simulink model "fullcar"  (Simulink 9.1)
settings: Solver=ode45  StartTime=0.0  StopTime=100  RelTol=1e-3  EnableMultiTasking=on
undefined symbols (not defined in the file): a, b, c_1, c_2, c_3, c_4, c_p, c_t, F_1, F_2, F_3, F_4, I_x, I_y, k_1, k_2, k_3, k_4, k_p, k_t, M, m_1, m_2, m_3, m_4, m_p, sigbuilder_block, w, x_p, y_p
settings Model: Creator=Zhytenko_Olexandr  LastModifiedBy=Saurabh Suman
settings SolverCC: MaxConsecutiveZCs=auto
settings DataIOCC: SignalLoggingSaveFormat=ModelDataLogs
settings OptimizationCC: BlockReduction=off  OptimizeBlockIOStorage=off  BufferReuse=off  GlobalBufferReuse=off  ExpressionFolding=off  ExpressionDepthLimit=2147483647  LocalBlockOutputs=off  OptimizeDataStoreBuffers=off  BusAssignmentInplaceUpdate=off
settings DebuggingCC: FcnCallInpInsideContextMsg=warning  StateNameClashWarn=warning
settings GRTTargetCC: GeneratePreprocessorConditionals=Disable all

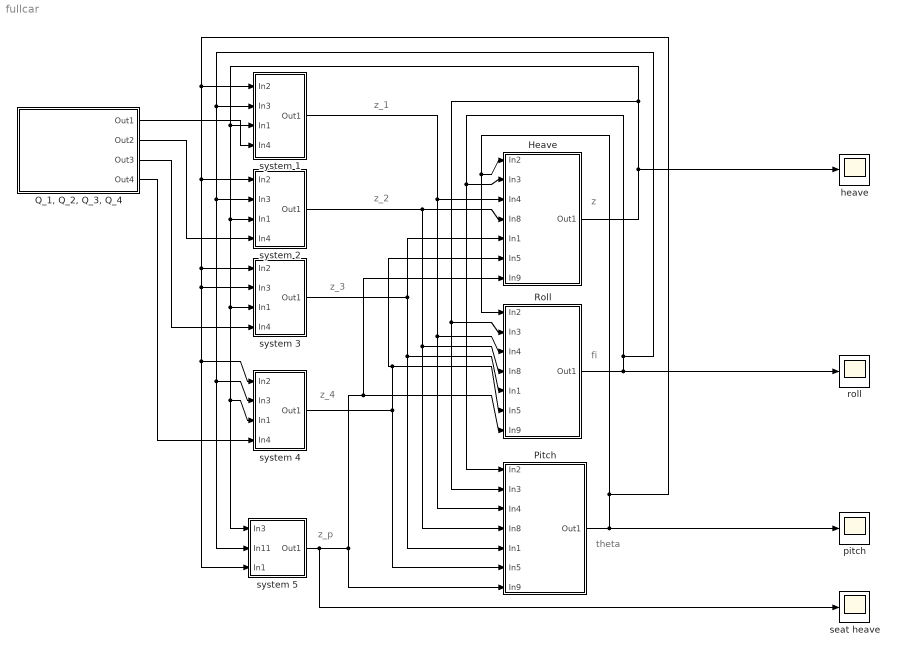
== system fullcar ==
  note: z
  note: fi
  note: theta
  note: z_p
  note: z_1
  note: z_2
  note: z_3
  note: z_4
  Heave : Subsystem
  Pitch : Subsystem
  "Q_1, Q_2, Q_3, Q_4" : Subsystem
  Roll : Subsystem
  heave : Scope
  pitch : Scope
  roll : Scope
  seat heave : Scope
  system 1 : Subsystem
  system 2 : Subsystem
  system 3 : Subsystem
  system 4 : Subsystem
  system 5 : Subsystem
  wires:
  Pitch/1(Out1) -> Heave/1(In2), Roll/1(In2), system 1/1(In2), system 2/1(In2), system 3/1(In2), system 3/2(In3), system 5/3(In1), system 4/1(In2), pitch/1
  Roll/1(Out1) -> Heave/2(In3), Pitch/1(In2), system 1/2(In3), system 2/2(In3), system 5/2(In11), system 4/2(In3), roll/1
  Heave/1(Out1) -> Roll/2(In3), Pitch/2(In3), system 1/3(In1), system 2/3(In1), system 3/3(In1), system 5/1(In3), system 4/3(In1), heave/1
  system 1/1(Out1) -> Heave/3(In4), Roll/3(In4), Pitch/3(In4)
  system 2/1(Out1) -> Heave/4(In8), Roll/4(In8), Pitch/4(In8)
  system 3/1(Out1) -> Heave/5(In1), Roll/5(In1), Pitch/5(In1)
  system 5/1(Out1) -> Heave/7(In9), Roll/7(In9), Pitch/7(In9), seat heave/1
  "Q_1, Q_2, Q_3, Q_4"/1(Out1) -> system 1/4(In4)
  "Q_1, Q_2, Q_3, Q_4"/2(Out2) -> system 2/4(In4)
  "Q_1, Q_2, Q_3, Q_4"/3(Out3) -> system 3/4(In4)
  "Q_1, Q_2, Q_3, Q_4"/4(Out4) -> system 4/4(In4)
  system 4/1(Out1) -> Heave/6(In5), Roll/6(In5), Pitch/6(In5)

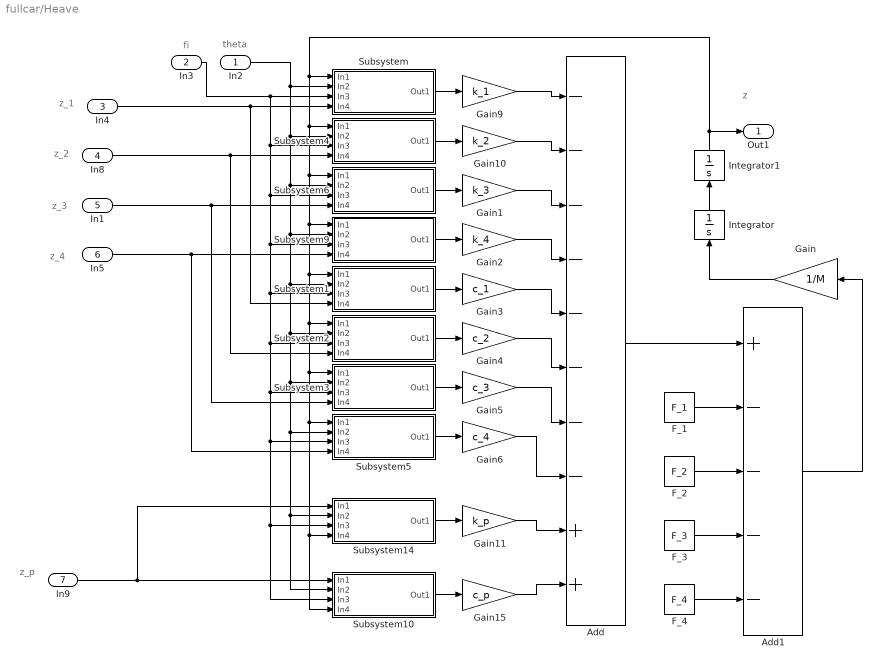
== system fullcar/Heave ==
  note: theta
  note: z
  note: fi
  note: z_1
  note: z_2
  note: z_3
  note: z_4
  note: z_p
  In2 : Inport
  In3 : Inport  Port=2
  In4 : Inport  Port=3
  In8 : Inport  Port=4
  In1 : Inport  Port=5
  In5 : Inport  Port=6
  In9 : Inport  Port=7
  Add : Sum  Inputs=--------++
  Add1 : Sum  Inputs=+----
  F_1 : Constant  Value=F_1
  F_2 : Constant  Value=F_2
  F_3 : Constant  Value=F_3
  F_4 : Constant  Value=F_4
  Gain : Gain  Gain=1/M
  Gain1 : Gain  Gain=k_3
  Gain10 : Gain  Gain=k_2
  Gain11 : Gain  Gain=k_p
  Gain15 : Gain  Gain=c_p
  Gain2 : Gain  Gain=k_4
  Gain3 : Gain  Gain=c_1
  Gain4 : Gain  Gain=c_2
  Gain5 : Gain  Gain=c_3
  Gain6 : Gain  Gain=c_4
  Gain9 : Gain  Gain=k_1
  Integrator : Integrator
  Integrator1 : Integrator
  Subsystem : Subsystem
  Subsystem1 : Subsystem
  Subsystem10 : Subsystem
  Subsystem14 : Subsystem
  Subsystem2 : Subsystem
  Subsystem3 : Subsystem
  Subsystem4 : Subsystem
  Subsystem5 : Subsystem
  Subsystem6 : Subsystem
  Subsystem9 : Subsystem
  Out1 : Outport
  wires:
  Gain10/1 -> Add/2
  Gain1/1 -> Add/3
  Gain2/1 -> Add/4
  Subsystem/1(Out1) -> Gain9/1
  Gain3/1 -> Add/5
  Gain4/1 -> Add/6
  Gain5/1 -> Add/7
  Subsystem1/1(Out1) -> Gain3/1
  Subsystem4/1(Out1) -> Gain10/1
  Subsystem2/1(Out1) -> Gain4/1
  Subsystem6/1(Out1) -> Gain1/1
  Subsystem3/1(Out1) -> Gain5/1
  Subsystem9/1(Out1) -> Gain2/1
  Subsystem5/1(Out1) -> Gain6/1
  Gain/1 -> Integrator/1
  Integrator/1 -> Integrator1/1
  Integrator1/1 -> Subsystem/1(In1), Subsystem4/1(In1), Subsystem6/1(In1), Subsystem9/1(In1), Subsystem1/1(In1), Subsystem2/1(In1), Subsystem3/1(In1), Subsystem5/1(In1), Subsystem10/4(In4), Subsystem14/4(In4), Out1/1
  Subsystem14/1(Out1) -> Gain11/1
  Subsystem10/1(Out1) -> Gain15/1
  In2/1 -> Subsystem/2(In2), Subsystem4/2(In2), Subsystem6/2(In2), Subsystem9/2(In2), Subsystem1/2(In2), Subsystem2/2(In2), Subsystem3/2(In2), Subsystem5/2(In2), Subsystem10/2(In2), Subsystem14/2(In2)
  In3/1 -> Subsystem/3(In3), Subsystem4/3(In3), Subsystem6/3(In3), Subsystem9/3(In3), Subsystem1/3(In3), Subsystem2/3(In3), Subsystem3/3(In3), Subsystem5/3(In3), Subsystem10/3(In3), Subsystem14/3(In3)
  In4/1 -> Subsystem/4(In4), Subsystem1/4(In4)
  In8/1 -> Subsystem4/4(In4), Subsystem2/4(In4)
  In1/1 -> Subsystem6/4(In4), Subsystem3/4(In4)
  In5/1 -> Subsystem9/4(In4), Subsystem5/4(In4)
  In9/1 -> Subsystem10/1(In1), Subsystem14/1(In1)
  Gain9/1 -> Add/1
  Gain15/1 -> Add/10
  Gain6/1 -> Add/8
  Gain11/1 -> Add/9
  Add/1 -> Add1/1
  F_1/1 -> Add1/2
  F_2/1 -> Add1/3
  F_3/1 -> Add1/4
  F_4/1 -> Add1/5
  Add1/1 -> Gain/1

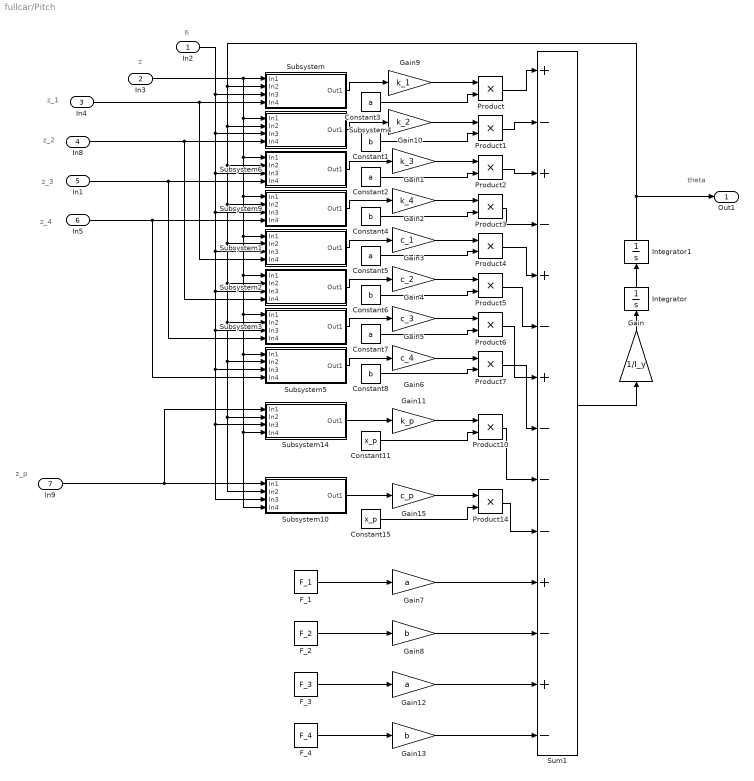
== system fullcar/Pitch ==
  note: fi
  note: theta
  note: z
  note: z_1
  note: z_2
  note: z_3
  note: z_4
  note: z_p
  In2 : Inport
  In3 : Inport  Port=2
  In4 : Inport  Port=3
  In8 : Inport  Port=4
  In1 : Inport  Port=5
  In5 : Inport  Port=6
  In9 : Inport  Port=7
  Constant{1,4,6,8} (4 alike) : Constant  Value=b
  Constant11 : Constant  Value=x_p
  Constant15 : Constant  Value=x_p
  Constant{2..3,5,7} (4 alike) : Constant  Value=a
  F_1 : Constant  Value=F_1
  F_2 : Constant  Value=F_2
  F_3 : Constant  Value=F_3
  F_4 : Constant  Value=F_4
  Gain : Gain  Gain=1/I_y
  Gain1 : Gain  Gain=k_3
  Gain10 : Gain  Gain=k_2
  Gain11 : Gain  Gain=k_p
  Gain12 : Gain  Gain=a
  Gain13 : Gain  Gain=b
  Gain15 : Gain  Gain=c_p
  Gain2 : Gain  Gain=k_4
  Gain3 : Gain  Gain=c_1
  Gain4 : Gain  Gain=c_2
  Gain5 : Gain  Gain=c_3
  Gain6 : Gain  Gain=c_4
  Gain7 : Gain  Gain=a
  Gain8 : Gain  Gain=b
  Gain9 : Gain  Gain=k_1
  Integrator : Integrator
  Integrator1 : Integrator
  Product{,1..7,10,14} (10 alike) : Product  RndMeth=Zero
  Subsystem : Subsystem
  Subsystem1 : Subsystem
  Subsystem10 : Subsystem
  Subsystem14 : Subsystem
  Subsystem2 : Subsystem
  Subsystem3 : Subsystem
  Subsystem4 : Subsystem
  Subsystem5 : Subsystem
  Subsystem6 : Subsystem
  Subsystem9 : Subsystem
  Sum1 : Sum  Inputs=+-+-+-+---+-+-
  Out1 : Outport
  wires:
  In3/1 -> Subsystem5/1(In1), Subsystem10/4(In4), Subsystem14/4(In4), Subsystem3/1(In1), Subsystem2/1(In1), Subsystem1/1(In1), Subsystem9/1(In1), Subsystem6/1(In1), Subsystem4/1(In1), Subsystem/1(In1)
  Constant15/1 -> Product14/2
  Gain15/1 -> Product14/1
  Constant11/1 -> Product10/2
  Gain11/1 -> Product10/1
  Constant8/1 -> Product7/2
  Subsystem5/1(Out1) -> Gain6/1
  Gain6/1 -> Product7/1
  Constant7/1 -> Product6/2
  Subsystem3/1(Out1) -> Gain5/1
  Gain5/1 -> Product6/1
  Constant6/1 -> Product5/2
  Subsystem2/1(Out1) -> Gain4/1
  Gain4/1 -> Product5/1
  Constant5/1 -> Product4/2
  Subsystem1/1(Out1) -> Gain3/1
  Gain3/1 -> Product4/1
  Constant4/1 -> Product3/2
  Subsystem9/1(Out1) -> Gain2/1
  Gain2/1 -> Product3/1
  Constant2/1 -> Product2/2
  Gain1/1 -> Product2/1
  Constant1/1 -> Product1/2
  Gain10/1 -> Product1/1
  Constant3/1 -> Product/2
  Gain9/1 -> Product/1
  Subsystem/1(Out1) -> Gain9/1
  Subsystem4/1(Out1) -> Gain10/1
  Subsystem6/1(Out1) -> Gain1/1
  Gain/1 -> Integrator/1
  Integrator/1 -> Integrator1/1
  Integrator1/1 -> Out1/1, Subsystem/2(In2), Subsystem4/2(In2), Subsystem6/2(In2), Subsystem9/2(In2), Subsystem1/2(In2), Subsystem2/2(In2), Subsystem3/2(In2), Subsystem5/2(In2), Subsystem10/2(In2), Subsystem14/2(In2)
  Subsystem14/1(Out1) -> Gain11/1
  Subsystem10/1(Out1) -> Gain15/1
  In4/1 -> Subsystem/4(In4), Subsystem1/4(In4)
  In8/1 -> Subsystem4/4(In4), Subsystem2/4(In4)
  In1/1 -> Subsystem6/4(In4), Subsystem3/4(In4)
  In5/1 -> Subsystem9/4(In4), Subsystem5/4(In4)
  In9/1 -> Subsystem10/1(In1), Subsystem14/1(In1)
  In2/1 -> Subsystem/3(In3), Subsystem4/3(In3), Subsystem6/3(In3), Subsystem9/3(In3), Subsystem1/3(In3), Subsystem2/3(In3), Subsystem3/3(In3), Subsystem5/3(In3), Subsystem10/3(In3), Subsystem14/3(In3)
  Product/1 -> Sum1/1
  Product1/1 -> Sum1/2
  Product2/1 -> Sum1/3
  Product3/1 -> Sum1/4
  Product4/1 -> Sum1/5
  Product5/1 -> Sum1/6
  Product6/1 -> Sum1/7
  Product7/1 -> Sum1/8
  Product10/1 -> Sum1/9
  Product14/1 -> Sum1/10
  F_1/1 -> Gain7/1
  F_2/1 -> Gain8/1
  F_3/1 -> Gain12/1
  F_4/1 -> Gain13/1
  Gain7/1 -> Sum1/11
  Gain8/1 -> Sum1/12
  Gain12/1 -> Sum1/13
  Gain13/1 -> Sum1/14
  Sum1/1 -> Gain/1

== system fullcar/Q_1, Q_2, Q_3, Q_4 ==
  note: Q_1
  note: Q_2
  note: Q_3
  note: Q_4
  Signal Builder : Subsystem  Tag=STV Subsys  LoadFcn=sigbuilder_block('load');  StartFcn=sigbuilder_block('start');  StopFcn=sigbuilder_block('stop');  ClipboardFcn=sigbuilder_block('clipboard');  mask(Sigbuilder block){tuvar=[0:10]}
      mask help: Create and generate interchangeable groups of signals whose waveforms are piecewise linear.
      mask init:
      | if ~strcmp(get_param(bdroot(gcbh),'SimulationStatus'),'stopped') tuvar = sigbuilder_block('maskInit'); end
      settings: CopyFcn=sigbuilder_block('copy');  DeleteFcn=sigbuilder_block('delete');  ModelCloseFcn=sigbuilder_block('modelClose');  PreSaveFcn=sigbuilder_block('preSave');  PauseFcn=sigbuilder_block('pause')  ContinueFcn=sigbuilder_block('continue')  NameChangeFcn=sigbuilder_block('namechange');  OpenFcn=sigbuilder_block('open',[437.25 118.5 550.5 394.5 ]);  CloseFcn=sigbuilder_block('close');
      mask Display: plot(0, 0, 100, 100,[2, 2, 32, 32, 2], [68, 8, 8, 68, 68],[32, 2], [38, 38], [32, 19, 2],[53, 60, 44], [32, 17, 17, 2],[16, 16, 31, 31]);txt = getActiveGroup(gcbh);text(2, 100, txt,'verticalAlignment', 'top');
  Transport Delay1 : TransportDelay  DelayTime=0.27
  Transport Delay2 : TransportDelay  DelayTime=0.27
  Out1 : Outport
  Out2 : Outport  Port=2
  Out3 : Outport  Port=3
  Out4 : Outport  Port=4
  wires:
  Signal Builder/1(Signal 1) -> Out1/1, Transport Delay1/1, Out3/1, Transport Delay2/1
  Transport Delay1/1 -> Out2/1
  Transport Delay2/1 -> Out4/1

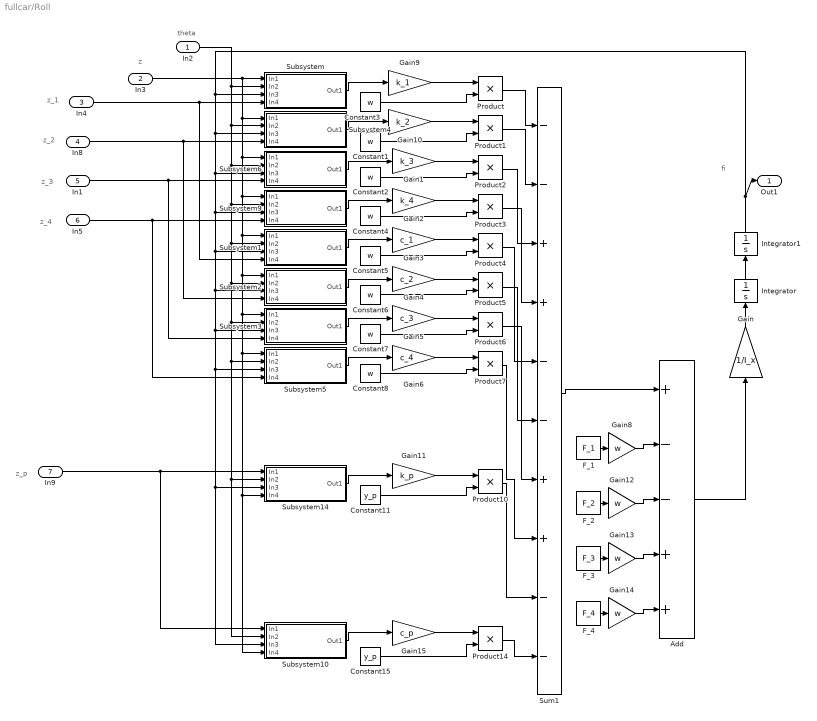
== system fullcar/Roll ==
  note: z_p
  note: z_4
  note: z_3
  note: z_2
  note: z_1
  note: z
  note: fi
  note: theta
  In2 : Inport
  In3 : Inport  Port=2
  In4 : Inport  Port=3
  In8 : Inport  Port=4
  In1 : Inport  Port=5
  In5 : Inport  Port=6
  In9 : Inport  Port=7
  Add : Sum  Inputs=+--++
  Constant{1..8} (8 alike) : Constant  Value=w
  Constant11 : Constant  Value=y_p
  Constant15 : Constant  Value=y_p
  F_1 : Constant  Value=F_1
  F_2 : Constant  Value=F_2
  F_3 : Constant  Value=F_3
  F_4 : Constant  Value=F_4
  Gain : Gain  Gain=1/I_x
  Gain1 : Gain  Gain=k_3
  Gain10 : Gain  Gain=k_2
  Gain11 : Gain  Gain=k_p
  Gain{8,12..14} (4 alike) : Gain  Gain=w
  Gain15 : Gain  Gain=c_p
  Gain2 : Gain  Gain=k_4
  Gain3 : Gain  Gain=c_1
  Gain4 : Gain  Gain=c_2
  Gain5 : Gain  Gain=c_3
  Gain6 : Gain  Gain=c_4
  Gain9 : Gain  Gain=k_1
  Integrator : Integrator  IgnoreLimit=on
  Integrator1 : Integrator
  Product{,1..7,10,14} (10 alike) : Product  RndMeth=Zero
  Subsystem : Subsystem
  Subsystem1 : Subsystem
  Subsystem10 : Subsystem
  Subsystem14 : Subsystem
  Subsystem2 : Subsystem
  Subsystem3 : Subsystem
  Subsystem4 : Subsystem
  Subsystem5 : Subsystem
  Subsystem6 : Subsystem
  Subsystem9 : Subsystem
  Sum1 : Sum  Inputs=--++--++--
  Out1 : Outport
  wires:
  In9/1 -> Subsystem10/1(In1), Subsystem14/1(In1)
  In5/1 -> Subsystem5/4(In4), Subsystem9/4(In4)
  In1/1 -> Subsystem3/4(In4), Subsystem6/4(In4)
  In8/1 -> Subsystem2/4(In4), Subsystem4/4(In4)
  In4/1 -> Subsystem1/4(In4), Subsystem/4(In4)
  In2/1 -> Subsystem5/2(In2), Subsystem14/2(In2), Subsystem10/2(In2), Subsystem3/2(In2), Subsystem2/2(In2), Subsystem1/2(In2), Subsystem9/2(In2), Subsystem6/2(In2), Subsystem4/2(In2), Subsystem/2(In2)
  Subsystem10/1(Out1) -> Gain15/1
  Subsystem14/1(Out1) -> Gain11/1
  Integrator1/1 -> Out1/1, Subsystem/3(In3), Subsystem4/3(In3), Subsystem6/3(In3), Subsystem9/3(In3), Subsystem1/3(In3), Subsystem2/3(In3), Subsystem3/3(In3), Subsystem5/3(In3), Subsystem14/3(In3), Subsystem10/3(In3)
  Integrator/1 -> Integrator1/1
  Gain/1 -> Integrator/1
  Subsystem6/1(Out1) -> Gain1/1
  Subsystem4/1(Out1) -> Gain10/1
  Subsystem/1(Out1) -> Gain9/1
  Product/1 -> Sum1/1
  Product1/1 -> Sum1/2
  Product2/1 -> Sum1/3
  Product3/1 -> Sum1/4
  Product4/1 -> Sum1/5
  Product5/1 -> Sum1/6
  Gain9/1 -> Product/1
  Constant3/1 -> Product/2
  Gain10/1 -> Product1/1
  Constant1/1 -> Product1/2
  Gain1/1 -> Product2/1
  Constant2/1 -> Product2/2
  Gain2/1 -> Product3/1
  Subsystem9/1(Out1) -> Gain2/1
  Constant4/1 -> Product3/2
  Gain3/1 -> Product4/1
  Subsystem1/1(Out1) -> Gain3/1
  Constant5/1 -> Product4/2
  Gain4/1 -> Product5/1
  Subsystem2/1(Out1) -> Gain4/1
  Constant6/1 -> Product5/2
  Gain5/1 -> Product6/1
  Subsystem3/1(Out1) -> Gain5/1
  Constant7/1 -> Product6/2
  Gain6/1 -> Product7/1
  Subsystem5/1(Out1) -> Gain6/1
  Constant8/1 -> Product7/2
  Gain11/1 -> Product10/1
  Constant11/1 -> Product10/2
  Gain15/1 -> Product14/1
  Constant15/1 -> Product14/2
  In3/1 -> Subsystem/1(In1), Subsystem4/1(In1), Subsystem6/1(In1), Subsystem9/1(In1), Subsystem1/1(In1), Subsystem2/1(In1), Subsystem3/1(In1), Subsystem5/1(In1), Subsystem14/4(In4), Subsystem10/4(In4)
  Sum1/1 -> Add/1
  Add/1 -> Gain/1
  F_1/1 -> Gain8/1
  Gain8/1 -> Add/2
  F_2/1 -> Gain12/1
  Gain12/1 -> Add/3
  F_3/1 -> Gain13/1
  Gain13/1 -> Add/4
  F_4/1 -> Gain14/1
  Gain14/1 -> Add/5
  Product6/1 -> Sum1/7
  Product7/1 -> Sum1/8
  Product10/1 -> Sum1/9
  Product14/1 -> Sum1/10

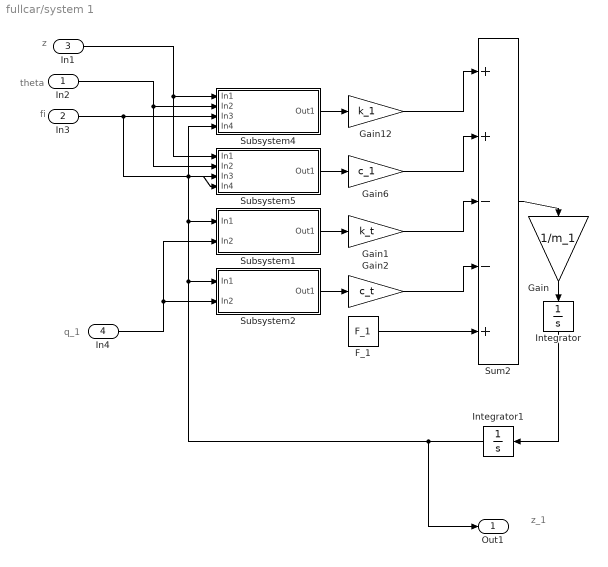
== system fullcar/system 1 ==
  note: fi
  note: z_1
  note: theta
  note: z
  note: q_1
  In2 : Inport
  In3 : Inport  Port=2
  In1 : Inport  Port=3
  In4 : Inport  Port=4
  F_1 : Constant  Value=F_1
  Gain : Gain  Gain=1/m_1
  Gain1 : Gain  Gain=k_t
  Gain12 : Gain  Gain=k_1
  Gain2 : Gain  Gain=c_t
  Gain6 : Gain  Gain=c_1
  Integrator : Integrator
  Integrator1 : Integrator
  Subsystem1 : Subsystem
  Subsystem2 : Subsystem
  Subsystem4 : Subsystem
  Subsystem5 : Subsystem
  Sum2 : Sum  Inputs=++--+
  Out1 : Outport
  wires:
  In3/1 -> Subsystem4/3(In3), Subsystem5/3(In3)
  In2/1 -> Subsystem4/2(In2), Subsystem5/2(In2)
  Integrator/1 -> Integrator1/1
  Gain/1 -> Integrator/1
  Gain6/1 -> Sum2/2
  Gain12/1 -> Sum2/1
  In1/1 -> Subsystem4/1(In1), Subsystem5/1(In1)
  Gain1/1 -> Sum2/3
  Gain2/1 -> Sum2/4
  Subsystem1/1(Out1) -> Gain1/1
  Subsystem2/1(Out1) -> Gain2/1
  Sum2/1 -> Gain/1
  Integrator1/1 -> Subsystem4/4(In4), Subsystem5/4(In4), Subsystem1/1(In1), Subsystem2/1(In1), Out1/1
  In4/1 -> Subsystem2/2(In2), Subsystem1/2(In2)
  Subsystem4/1(Out1) -> Gain12/1
  Subsystem5/1(Out1) -> Gain6/1
  F_1/1 -> Sum2/5

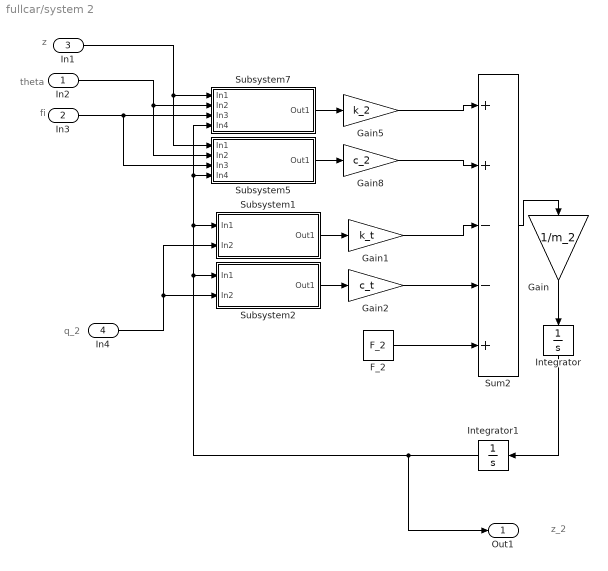
== system fullcar/system 2 ==
  note: q_2
  note: z
  note: theta
  note: z_2
  note: fi
  In2 : Inport
  In3 : Inport  Port=2
  In1 : Inport  Port=3
  In4 : Inport  Port=4
  F_2 : Constant  Value=F_2
  Gain : Gain  Gain=1/m_2
  Gain1 : Gain  Gain=k_t
  Gain2 : Gain  Gain=c_t
  Gain5 : Gain  Gain=k_2
  Gain8 : Gain  Gain=c_2
  Integrator : Integrator
  Integrator1 : Integrator
  Subsystem1 : Subsystem
  Subsystem2 : Subsystem
  Subsystem5 : Subsystem
  Subsystem7 : Subsystem
  Sum2 : Sum  Inputs=++--+
  Out1 : Outport
  wires:
  In4/1 -> Subsystem2/2(In2), Subsystem1/2(In2)
  Integrator1/1 -> Subsystem7/4(In4), Subsystem5/4(In4), Subsystem1/1(In1), Subsystem2/1(In1), Out1/1
  Subsystem2/1(Out1) -> Gain2/1
  Subsystem1/1(Out1) -> Gain1/1
  Gain2/1 -> Sum2/4
  Gain1/1 -> Sum2/3
  In1/1 -> Subsystem7/1(In1), Subsystem5/1(In1)
  Gain5/1 -> Sum2/1
  Gain8/1 -> Sum2/2
  In2/1 -> Subsystem7/2(In2), Subsystem5/2(In2)
  In3/1 -> Subsystem7/3(In3), Subsystem5/3(In3)
  Subsystem7/1(Out1) -> Gain5/1
  Subsystem5/1(Out1) -> Gain8/1
  F_2/1 -> Sum2/5
  Integrator/1 -> Integrator1/1
  Gain/1 -> Integrator/1
  Sum2/1 -> Gain/1

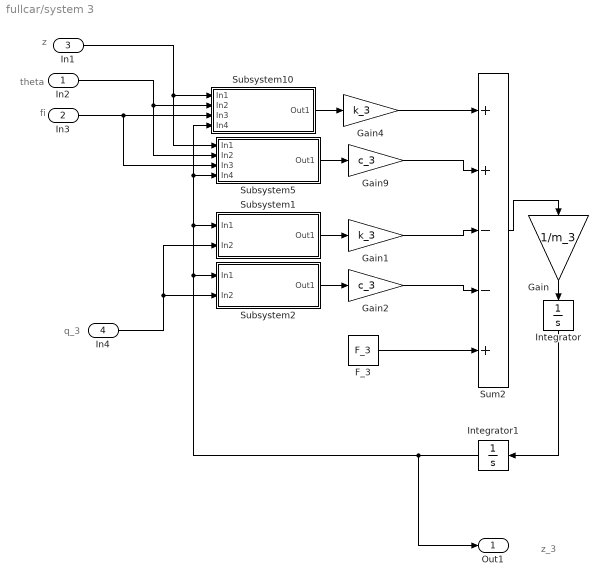
== system fullcar/system 3 ==
  note: fi
  note: z_3
  note: theta
  note: z
  note: q_3
  In2 : Inport
  In3 : Inport  Port=2
  In1 : Inport  Port=3
  In4 : Inport  Port=4
  F_3 : Constant  Value=F_3
  Gain : Gain  Gain=1/m_3
  Gain1 : Gain  Gain=k_3
  Gain2 : Gain  Gain=c_3
  Gain4 : Gain  Gain=k_3
  Gain9 : Gain  Gain=c_3
  Integrator : Integrator
  Integrator1 : Integrator
  Subsystem1 : Subsystem
  Subsystem10 : Subsystem
  Subsystem2 : Subsystem
  Subsystem5 : Subsystem
  Sum2 : Sum  Inputs=++--+
  Out1 : Outport
  wires:
  In3/1 -> Subsystem10/3(In3), Subsystem5/3(In3)
  In2/1 -> Subsystem10/2(In2), Subsystem5/2(In2)
  Integrator/1 -> Integrator1/1
  Gain/1 -> Integrator/1
  Gain9/1 -> Sum2/2
  Gain4/1 -> Sum2/1
  In1/1 -> Subsystem10/1(In1), Subsystem5/1(In1)
  Gain1/1 -> Sum2/3
  Gain2/1 -> Sum2/4
  Subsystem1/1(Out1) -> Gain1/1
  Subsystem2/1(Out1) -> Gain2/1
  Sum2/1 -> Gain/1
  Integrator1/1 -> Subsystem2/1(In1), Subsystem1/1(In1), Subsystem10/4(In4), Subsystem5/4(In4), Out1/1
  In4/1 -> Subsystem1/2(In2), Subsystem2/2(In2)
  Subsystem10/1(Out1) -> Gain4/1
  Subsystem5/1(Out1) -> Gain9/1
  F_3/1 -> Sum2/5

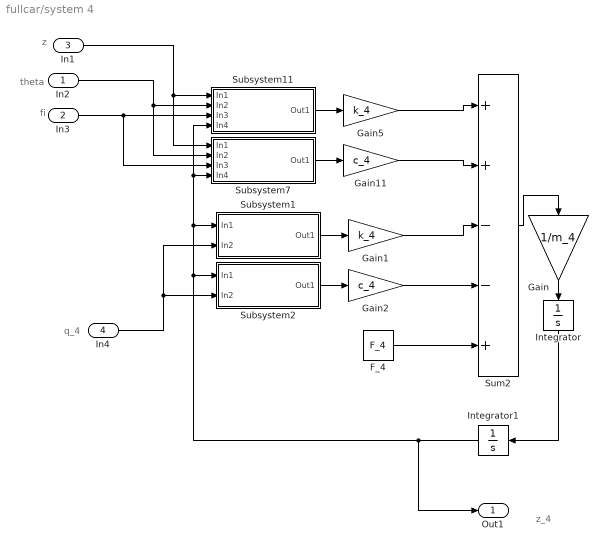
== system fullcar/system 4 ==
  note: q_4
  note: z
  note: theta
  note: z_4
  note: fi
  In2 : Inport
  In3 : Inport  Port=2
  In1 : Inport  Port=3
  In4 : Inport  Port=4
  F_4 : Constant  Value=F_4
  Gain : Gain  Gain=1/m_4
  Gain1 : Gain  Gain=k_4
  Gain11 : Gain  Gain=c_4
  Gain2 : Gain  Gain=c_4
  Gain5 : Gain  Gain=k_4
  Integrator : Integrator
  Integrator1 : Integrator
  Subsystem1 : Subsystem
  Subsystem11 : Subsystem
  Subsystem2 : Subsystem
  Subsystem7 : Subsystem
  Sum2 : Sum  Inputs=++--+
  Out1 : Outport
  wires:
  In4/1 -> Subsystem2/2(In2), Subsystem1/2(In2)
  Integrator1/1 -> Subsystem11/4(In4), Subsystem7/4(In4), Subsystem1/1(In1), Subsystem2/1(In1), Out1/1
  Sum2/1 -> Gain/1
  Subsystem2/1(Out1) -> Gain2/1
  Subsystem1/1(Out1) -> Gain1/1
  Gain2/1 -> Sum2/4
  Gain1/1 -> Sum2/3
  In1/1 -> Subsystem11/1(In1), Subsystem7/1(In1)
  Gain5/1 -> Sum2/1
  Gain11/1 -> Sum2/2
  Gain/1 -> Integrator/1
  Integrator/1 -> Integrator1/1
  In2/1 -> Subsystem11/2(In2), Subsystem7/2(In2)
  In3/1 -> Subsystem11/3(In3), Subsystem7/3(In3)
  Subsystem11/1(Out1) -> Gain5/1
  Subsystem7/1(Out1) -> Gain11/1
  F_4/1 -> Sum2/5

== system fullcar/system 5 ==
  note: fi
  note: z_3
  note: z
  note: theta
  In3 : Inport
  In11 : Inport  Port=2
  In1 : Inport  Port=3
  Gain : Gain  Gain=1/m_p
  Gain3 : Gain  Gain=k_p
  Gain4 : Gain  Gain=c_p
  Integrator : Integrator
  Integrator1 : Integrator
  Subsystem2 : Subsystem
  Subsystem3 : Subsystem
  Sum : Sum  Inputs=--
  Out1 : Outport
  wires:
  Integrator/1 -> Integrator1/1
  Gain/1 -> Integrator/1
  Sum/1 -> Gain/1
  Gain4/1 -> Sum/2
  Gain3/1 -> Sum/1
  In1/1 -> Subsystem2/2(In2), Subsystem3/2(In2)
  Integrator1/1 -> Out1/1, Subsystem2/1(In1), Subsystem3/1(In1)
  Subsystem2/1(Out1) -> Gain3/1
  Subsystem3/1(Out1) -> Gain4/1
  In11/1 -> Subsystem2/3(In3), Subsystem3/3(In3)
  In3/1 -> Subsystem2/4(In4), Subsystem3/4(In4)

== system fullcar/Heave/Subsystem ==
  note: z
  note: theta
  note: fi
  note: z_1
  In1 : Inport
  In2 : Inport  Port=2
  In3 : Inport  Port=3
  In4 : Inport  Port=4
  Constant : Constant  Value=a
  Constant1 : Constant  Value=w
  Product : Product  RndMeth=Zero
  Product1 : Product  RndMeth=Zero
  Sum : Sum  Inputs=+-+
  Sum1 : Sum  Inputs=+-
  Out1 : Outport
  wires:
  Sum1/1 -> Out1/1
  Sum/1 -> Sum1/1
  In4/1 -> Sum1/2
  In1/1 -> Sum/1
  In2/1 -> Product/1
  Constant/1 -> Product/2
  Product/1 -> Sum/2
  In3/1 -> Product1/1
  Constant1/1 -> Product1/2
  Product1/1 -> Sum/3

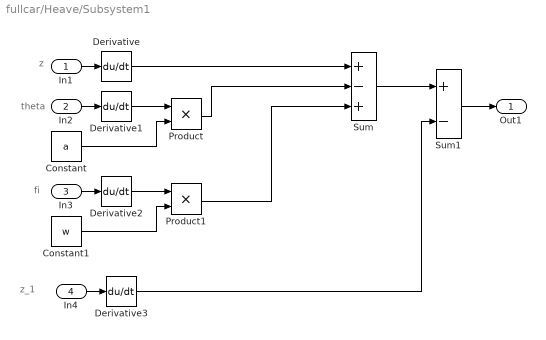
== system fullcar/Heave/Subsystem1 ==
  note: z_1
  note: fi
  note: theta
  note: z
  In1 : Inport
  In2 : Inport  Port=2
  In3 : Inport  Port=3
  In4 : Inport  Port=4
  Constant : Constant  Value=a
  Constant1 : Constant  Value=w
  Derivative{,1..3} (4 alike) : Derivative
  Product : Product  RndMeth=Zero
  Product1 : Product  RndMeth=Zero
  Sum : Sum  Inputs=+-+
  Sum1 : Sum  Inputs=+-
  Out1 : Outport
  wires:
  Product1/1 -> Sum/3
  Constant1/1 -> Product1/2
  In3/1 -> Derivative2/1
  Product/1 -> Sum/2
  Constant/1 -> Product/2
  In2/1 -> Derivative1/1
  In1/1 -> Derivative/1
  In4/1 -> Derivative3/1
  Sum/1 -> Sum1/1
  Sum1/1 -> Out1/1
  Derivative/1 -> Sum/1
  Derivative1/1 -> Product/1
  Derivative2/1 -> Product1/1
  Derivative3/1 -> Sum1/2

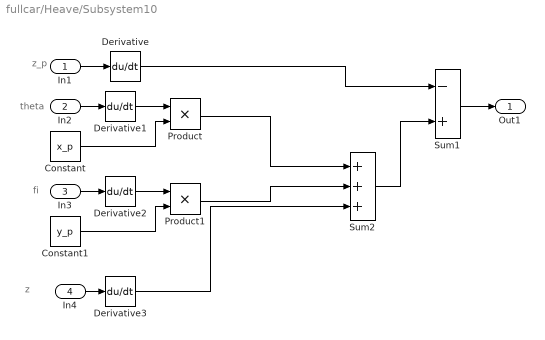
== system fullcar/Heave/Subsystem10 ==
  note: z_p
  note: theta
  note: fi
  note: z
  In1 : Inport
  In2 : Inport  Port=2
  In3 : Inport  Port=3
  In4 : Inport  Port=4
  Constant : Constant  Value=x_p
  Constant1 : Constant  Value=y_p
  Derivative{,1..3} (4 alike) : Derivative
  Product : Product  RndMeth=Zero
  Product1 : Product  RndMeth=Zero
  Sum1 : Sum  Inputs=-+
  Sum2 : Sum  Inputs=+++
  Out1 : Outport
  wires:
  Sum2/1 -> Sum1/2
  In4/1 -> Derivative3/1
  Product1/1 -> Sum2/2
  Product/1 -> Sum2/1
  In1/1 -> Derivative/1
  Sum1/1 -> Out1/1
  In2/1 -> Derivative1/1
  Constant/1 -> Product/2
  In3/1 -> Derivative2/1
  Constant1/1 -> Product1/2
  Derivative/1 -> Sum1/1
  Derivative1/1 -> Product/1
  Derivative2/1 -> Product1/1
  Derivative3/1 -> Sum2/3

== system fullcar/Heave/Subsystem14 ==
  note: z
  note: fi
  note: theta
  note: z_p
  In1 : Inport
  In2 : Inport  Port=2
  In3 : Inport  Port=3
  In4 : Inport  Port=4
  Constant : Constant  Value=x_p
  Constant1 : Constant  Value=y_p
  Product : Product  RndMeth=Zero
  Product1 : Product  RndMeth=Zero
  Sum1 : Sum  Inputs=-+
  Sum2 : Sum  Inputs=+++
  Out1 : Outport
  wires:
  Constant1/1 -> Product1/2
  In3/1 -> Product1/1
  Constant/1 -> Product/2
  In2/1 -> Product/1
  Sum1/1 -> Out1/1
  In1/1 -> Sum1/1
  Product/1 -> Sum2/1
  Product1/1 -> Sum2/2
  In4/1 -> Sum2/3
  Sum2/1 -> Sum1/2

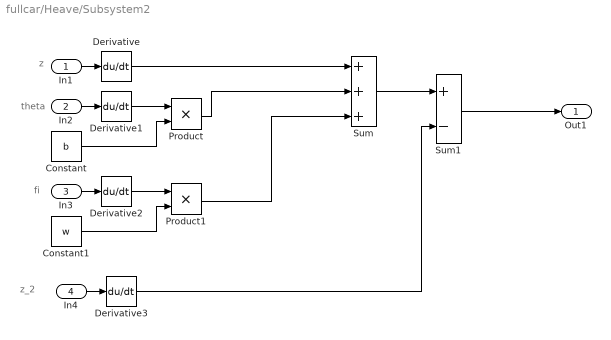
== system fullcar/Heave/Subsystem2 ==
  note: z
  note: theta
  note: fi
  note: z_2
  In1 : Inport
  In2 : Inport  Port=2
  In3 : Inport  Port=3
  In4 : Inport  Port=4
  Constant : Constant  Value=b
  Constant1 : Constant  Value=w
  Derivative{,1..3} (4 alike) : Derivative
  Product : Product  RndMeth=Zero
  Product1 : Product  RndMeth=Zero
  Sum : Sum  Inputs=+++
  Sum1 : Sum  Inputs=+-
  Out1 : Outport
  wires:
  Sum1/1 -> Out1/1
  Sum/1 -> Sum1/1
  In4/1 -> Derivative3/1
  In1/1 -> Derivative/1
  In2/1 -> Derivative1/1
  Constant/1 -> Product/2
  Product/1 -> Sum/2
  In3/1 -> Derivative2/1
  Constant1/1 -> Product1/2
  Product1/1 -> Sum/3
  Derivative/1 -> Sum/1
  Derivative1/1 -> Product/1
  Derivative2/1 -> Product1/1
  Derivative3/1 -> Sum1/2

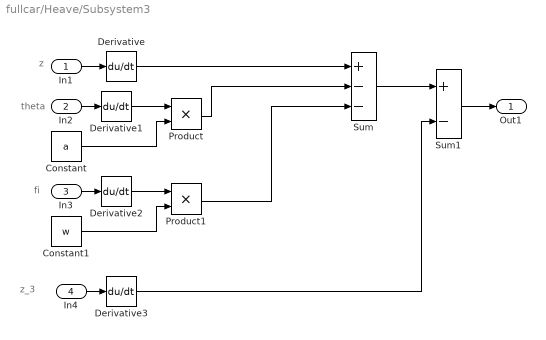
== system fullcar/Heave/Subsystem3 ==
  note: z_3
  note: fi
  note: theta
  note: z
  In1 : Inport
  In2 : Inport  Port=2
  In3 : Inport  Port=3
  In4 : Inport  Port=4
  Constant : Constant  Value=a
  Constant1 : Constant  Value=w
  Derivative{,1..3} (4 alike) : Derivative
  Product : Product  RndMeth=Zero
  Product1 : Product  RndMeth=Zero
  Sum : Sum  Inputs=+--
  Sum1 : Sum  Inputs=+-
  Out1 : Outport
  wires:
  Product1/1 -> Sum/3
  Constant1/1 -> Product1/2
  In3/1 -> Derivative2/1
  Product/1 -> Sum/2
  Constant/1 -> Product/2
  In2/1 -> Derivative1/1
  In1/1 -> Derivative/1
  In4/1 -> Derivative3/1
  Sum/1 -> Sum1/1
  Sum1/1 -> Out1/1
  Derivative/1 -> Sum/1
  Derivative1/1 -> Product/1
  Derivative2/1 -> Product1/1
  Derivative3/1 -> Sum1/2

== system fullcar/Heave/Subsystem4 ==
  note: z_2
  note: fi
  note: theta
  note: z
  In1 : Inport
  In2 : Inport  Port=2
  In3 : Inport  Port=3
  In4 : Inport  Port=4
  Constant : Constant  Value=b
  Constant1 : Constant  Value=w
  Product : Product  RndMeth=Zero
  Product1 : Product  RndMeth=Zero
  Sum : Sum  Inputs=+++
  Sum1 : Sum  Inputs=+-
  Out1 : Outport
  wires:
  Product1/1 -> Sum/3
  Constant1/1 -> Product1/2
  In3/1 -> Product1/1
  Product/1 -> Sum/2
  Constant/1 -> Product/2
  In2/1 -> Product/1
  In1/1 -> Sum/1
  In4/1 -> Sum1/2
  Sum1/1 -> Out1/1
  Sum/1 -> Sum1/1

== system fullcar/Heave/Subsystem5 ==
  note: z_4
  note: fi
  note: theta
  note: z
  In1 : Inport
  In2 : Inport  Port=2
  In3 : Inport  Port=3
  In4 : Inport  Port=4
  Constant : Constant  Value=b
  Constant1 : Constant  Value=w
  Derivative{,1..3} (4 alike) : Derivative
  Product : Product  RndMeth=Zero
  Product1 : Product  RndMeth=Zero
  Sum : Sum  Inputs=++-
  Sum1 : Sum  Inputs=+-
  Out1 : Outport
  wires:
  Product1/1 -> Sum/3
  Constant1/1 -> Product1/2
  In3/1 -> Derivative2/1
  Product/1 -> Sum/2
  Constant/1 -> Product/2
  In2/1 -> Derivative1/1
  In1/1 -> Derivative/1
  In4/1 -> Derivative3/1
  Sum/1 -> Sum1/1
  Sum1/1 -> Out1/1
  Derivative/1 -> Sum/1
  Derivative1/1 -> Product/1
  Derivative2/1 -> Product1/1
  Derivative3/1 -> Sum1/2

== system fullcar/Heave/Subsystem6 ==
  note: z
  note: theta
  note: fi
  note: z_3
  In1 : Inport
  In2 : Inport  Port=2
  In3 : Inport  Port=3
  In4 : Inport  Port=4
  Constant : Constant  Value=a
  Constant1 : Constant  Value=w
  Product : Product  RndMeth=Zero
  Product1 : Product  RndMeth=Zero
  Sum : Sum  Inputs=+--
  Sum1 : Sum  Inputs=+-
  Out1 : Outport
  wires:
  Sum1/1 -> Out1/1
  Sum/1 -> Sum1/1
  In4/1 -> Sum1/2
  In1/1 -> Sum/1
  In2/1 -> Product/1
  Constant/1 -> Product/2
  Product/1 -> Sum/2
  In3/1 -> Product1/1
  Constant1/1 -> Product1/2
  Product1/1 -> Sum/3

== system fullcar/Heave/Subsystem9 ==
  note: z
  note: theta
  note: fi
  note: z_4
  In1 : Inport
  In2 : Inport  Port=2
  In3 : Inport  Port=3
  In4 : Inport  Port=4
  Constant : Constant  Value=b
  Constant1 : Constant  Value=w
  Product : Product  RndMeth=Zero
  Product1 : Product  RndMeth=Zero
  Sum : Sum  Inputs=++-
  Sum1 : Sum  Inputs=+-
  Out1 : Outport
  wires:
  Sum1/1 -> Out1/1
  Sum/1 -> Sum1/1
  In4/1 -> Sum1/2
  In1/1 -> Sum/1
  In2/1 -> Product/1
  Constant/1 -> Product/2
  Product/1 -> Sum/2
  In3/1 -> Product1/1
  Constant1/1 -> Product1/2
  Product1/1 -> Sum/3

== system fullcar/Pitch/Subsystem ==
  note: z
  note: theta
  note: fi
  note: z_1
  In1 : Inport
  In2 : Inport  Port=2
  In3 : Inport  Port=3
  In4 : Inport  Port=4
  Constant : Constant  Value=a
  Constant1 : Constant  Value=w
  Product : Product  RndMeth=Zero
  Product1 : Product  RndMeth=Zero
  Sum : Sum  Inputs=++-
  Sum1 : Sum  Inputs=+-
  Out1 : Outport
  wires:
  Sum1/1 -> Out1/1
  Sum/1 -> Sum1/1
  In4/1 -> Sum1/2
  In1/1 -> Sum/1
  In2/1 -> Product/1
  Constant/1 -> Product/2
  Product/1 -> Sum/2
  In3/1 -> Product1/1
  Constant1/1 -> Product1/2
  Product1/1 -> Sum/3

== system fullcar/Pitch/Subsystem1 ==
  note: z_1
  note: fi
  note: theta
  note: z
  In1 : Inport
  In2 : Inport  Port=2
  In3 : Inport  Port=3
  In4 : Inport  Port=4
  Constant : Constant  Value=a
  Constant1 : Constant  Value=w
  Derivative{,1..3} (4 alike) : Derivative
  Product : Product  RndMeth=Zero
  Product1 : Product  RndMeth=Zero
  Sum : Sum  Inputs=++-
  Sum1 : Sum  Inputs=+-
  Out1 : Outport
  wires:
  Product1/1 -> Sum/3
  Constant1/1 -> Product1/2
  In3/1 -> Derivative2/1
  Product/1 -> Sum/2
  Constant/1 -> Product/2
  In2/1 -> Derivative1/1
  In1/1 -> Derivative/1
  In4/1 -> Derivative3/1
  Sum/1 -> Sum1/1
  Sum1/1 -> Out1/1
  Derivative/1 -> Sum/1
  Derivative1/1 -> Product/1
  Derivative2/1 -> Product1/1
  Derivative3/1 -> Sum1/2

== system fullcar/Pitch/Subsystem10 ==
  note: z_p
  note: theta
  note: fi
  note: z
  In1 : Inport
  In2 : Inport  Port=2
  In3 : Inport  Port=3
  In4 : Inport  Port=4
  Constant : Constant  Value=x_p
  Constant1 : Constant  Value=y_p
  Derivative{,1..3} (4 alike) : Derivative
  Product : Product  RndMeth=Zero
  Product1 : Product  RndMeth=Zero
  Sum1 : Sum
  Sum2 : Sum  Inputs=---
  Out1 : Outport
  wires:
  Sum2/1 -> Sum1/2
  In4/1 -> Derivative3/1
  Product1/1 -> Sum2/2
  Product/1 -> Sum2/1
  In1/1 -> Derivative/1
  Sum1/1 -> Out1/1
  In2/1 -> Derivative1/1
  Constant/1 -> Product/2
  In3/1 -> Derivative2/1
  Constant1/1 -> Product1/2
  Derivative/1 -> Sum1/1
  Derivative1/1 -> Product/1
  Derivative2/1 -> Product1/1
  Derivative3/1 -> Sum2/3

== system fullcar/Pitch/Subsystem14 ==
  note: z
  note: fi
  note: theta
  note: z_p
  In1 : Inport
  In2 : Inport  Port=2
  In3 : Inport  Port=3
  In4 : Inport  Port=4
  Constant : Constant  Value=x_p
  Constant1 : Constant  Value=y_p
  Product : Product  RndMeth=Zero
  Product1 : Product  RndMeth=Zero
  Sum1 : Sum
  Sum2 : Sum  Inputs=---
  Out1 : Outport
  wires:
  Constant1/1 -> Product1/2
  In3/1 -> Product1/1
  Constant/1 -> Product/2
  In2/1 -> Product/1
  Sum1/1 -> Out1/1
  In1/1 -> Sum1/1
  Product/1 -> Sum2/1
  Product1/1 -> Sum2/2
  In4/1 -> Sum2/3
  Sum2/1 -> Sum1/2

== system fullcar/Pitch/Subsystem2 ==
  note: z
  note: theta
  note: fi
  note: z_2
  In1 : Inport
  In2 : Inport  Port=2
  In3 : Inport  Port=3
  In4 : Inport  Port=4
  Constant : Constant  Value=b
  Constant1 : Constant  Value=w
  Derivative{,1..3} (4 alike) : Derivative
  Product : Product  RndMeth=Zero
  Product1 : Product  RndMeth=Zero
  Sum : Sum  Inputs=+++
  Sum1 : Sum  Inputs=+-
  Out1 : Outport
  wires:
  Sum1/1 -> Out1/1
  Sum/1 -> Sum1/1
  In4/1 -> Derivative3/1
  In1/1 -> Derivative/1
  In2/1 -> Derivative1/1
  Constant/1 -> Product/2
  Product/1 -> Sum/2
  In3/1 -> Derivative2/1
  Constant1/1 -> Product1/2
  Product1/1 -> Sum/3
  Derivative/1 -> Sum/1
  Derivative1/1 -> Product/1
  Derivative2/1 -> Product1/1
  Derivative3/1 -> Sum1/2

== system fullcar/Pitch/Subsystem3 ==
  note: z_3
  note: fi
  note: theta
  note: z
  In1 : Inport
  In2 : Inport  Port=2
  In3 : Inport  Port=3
  In4 : Inport  Port=4
  Constant : Constant  Value=a
  Constant1 : Constant  Value=w
  Derivative{,1..3} (4 alike) : Derivative
  Product : Product  RndMeth=Zero
  Product1 : Product  RndMeth=Zero
  Sum : Sum  Inputs=+++
  Sum1 : Sum  Inputs=+-
  Out1 : Outport
  wires:
  Product1/1 -> Sum/3
  Constant1/1 -> Product1/2
  In3/1 -> Derivative2/1
  Product/1 -> Sum/2
  Constant/1 -> Product/2
  In2/1 -> Derivative1/1
  In1/1 -> Derivative/1
  In4/1 -> Derivative3/1
  Sum/1 -> Sum1/1
  Sum1/1 -> Out1/1
  Derivative/1 -> Sum/1
  Derivative1/1 -> Product/1
  Derivative2/1 -> Product1/1
  Derivative3/1 -> Sum1/2

== system fullcar/Pitch/Subsystem4 ==
  note: z_2
  note: fi
  note: theta
  note: z
  In1 : Inport
  In2 : Inport  Port=2
  In3 : Inport  Port=3
  In4 : Inport  Port=4
  Constant : Constant  Value=b
  Constant1 : Constant  Value=w
  Product : Product  RndMeth=Zero
  Product1 : Product  RndMeth=Zero
  Sum : Sum  Inputs=+++
  Sum1 : Sum  Inputs=+-
  Out1 : Outport
  wires:
  Product1/1 -> Sum/3
  Constant1/1 -> Product1/2
  In3/1 -> Product1/1
  Product/1 -> Sum/2
  Constant/1 -> Product/2
  In2/1 -> Product/1
  In1/1 -> Sum/1
  In4/1 -> Sum1/2
  Sum/1 -> Sum1/1
  Sum1/1 -> Out1/1

== system fullcar/Pitch/Subsystem5 ==
  note: z_4
  note: fi
  note: theta
  note: z
  In1 : Inport
  In2 : Inport  Port=2
  In3 : Inport  Port=3
  In4 : Inport  Port=4
  Constant : Constant  Value=b
  Constant1 : Constant  Value=w
  Derivative{,1..3} (4 alike) : Derivative
  Product : Product  RndMeth=Zero
  Product1 : Product  RndMeth=Zero
  Sum : Sum  Inputs=++-
  Sum1 : Sum  Inputs=+-
  Out1 : Outport
  wires:
  Product1/1 -> Sum/3
  Constant1/1 -> Product1/2
  In3/1 -> Derivative2/1
  Product/1 -> Sum/2
  Constant/1 -> Product/2
  In2/1 -> Derivative1/1
  In1/1 -> Derivative/1
  In4/1 -> Derivative3/1
  Sum/1 -> Sum1/1
  Sum1/1 -> Out1/1
  Derivative/1 -> Sum/1
  Derivative1/1 -> Product/1
  Derivative2/1 -> Product1/1
  Derivative3/1 -> Sum1/2

== system fullcar/Pitch/Subsystem6 ==
  note: z
  note: theta
  note: fi
  note: z_3
  In1 : Inport
  In2 : Inport  Port=2
  In3 : Inport  Port=3
  In4 : Inport  Port=4
  Constant : Constant  Value=a
  Constant1 : Constant  Value=w
  Product : Product  RndMeth=Zero
  Product1 : Product  RndMeth=Zero
  Sum : Sum  Inputs=+++
  Sum1 : Sum  Inputs=+-
  Out1 : Outport
  wires:
  Sum1/1 -> Out1/1
  Sum/1 -> Sum1/1
  In4/1 -> Sum1/2
  In1/1 -> Sum/1
  In2/1 -> Product/1
  Constant/1 -> Product/2
  Product/1 -> Sum/2
  In3/1 -> Product1/1
  Constant1/1 -> Product1/2
  Product1/1 -> Sum/3

== system fullcar/Pitch/Subsystem9 ==
  note: z
  note: theta
  note: fi
  note: z_4
  In1 : Inport
  In2 : Inport  Port=2
  In3 : Inport  Port=3
  In4 : Inport  Port=4
  Constant : Constant  Value=b
  Constant1 : Constant  Value=w
  Product : Product  RndMeth=Zero
  Product1 : Product  RndMeth=Zero
  Sum : Sum  Inputs=++-
  Sum1 : Sum  Inputs=+-
  Out1 : Outport
  wires:
  Sum1/1 -> Out1/1
  Sum/1 -> Sum1/1
  In4/1 -> Sum1/2
  In1/1 -> Sum/1
  In2/1 -> Product/1
  Constant/1 -> Product/2
  Product/1 -> Sum/2
  In3/1 -> Product1/1
  Constant1/1 -> Product1/2
  Product1/1 -> Sum/3

== system fullcar/Q_1, Q_2, Q_3, Q_4/Signal Builder ==
  Demux : Demux  Tag=STV Demux  Outputs=1
  FromWs : FromWorkspace  Tag=STV FromWs  VariableName=tuvar  SampleTime=0  SigBuilderData=DataTag0  VnvData=DataTag1
      SigBuilderData=|
      | common.afterFinalStr = 'Extrapolate'
      | common.sampleTime = 0
      | dataSet.timeRange = [0 10]
      | dataSet.name = 'Group 1'
      | sbobj.Groups.Name = 'Group 1'
      | sbobj.Groups.Signals.Name = 'Signal 1'
      | sbobj.Groups.Signals.XData = [0 4 4 6 6 10]
      | sbobj.Groups.Signals.YData = [0 0 1 1 0 0]
  Signal 1 : Outport  Tag=STV Outport
  wires:
  Demux/1 -> Signal 1/1
  FromWs/1 -> Demux/1

== system fullcar/Roll/Subsystem ==
  note: z_1
  note: fi
  note: theta
  note: z
  In1 : Inport
  In2 : Inport  Port=2
  In3 : Inport  Port=3
  In4 : Inport  Port=4
  Constant : Constant  Value=a
  Constant1 : Constant  Value=w
  Product : Product  RndMeth=Zero
  Product1 : Product  RndMeth=Zero
  Sum : Sum  Inputs=+-+
  Sum1 : Sum  Inputs=+-
  Out1 : Outport
  wires:
  Product1/1 -> Sum/3
  Constant1/1 -> Product1/2
  In3/1 -> Product1/1
  Product/1 -> Sum/2
  Constant/1 -> Product/2
  In2/1 -> Product/1
  In1/1 -> Sum/1
  In4/1 -> Sum1/2
  Sum/1 -> Sum1/1
  Sum1/1 -> Out1/1

== system fullcar/Roll/Subsystem1 ==
  note: z
  note: theta
  note: fi
  note: z_1
  In1 : Inport
  In2 : Inport  Port=2
  In3 : Inport  Port=3
  In4 : Inport  Port=4
  Constant : Constant  Value=a
  Constant1 : Constant  Value=w
  Derivative{,1..3} (4 alike) : Derivative
  Product : Product  RndMeth=Zero
  Product1 : Product  RndMeth=Zero
  Sum : Sum  Inputs=+-+
  Sum1 : Sum  Inputs=+-
  Out1 : Outport
  wires:
  Derivative3/1 -> Sum1/2
  Derivative2/1 -> Product1/1
  Derivative1/1 -> Product/1
  Derivative/1 -> Sum/1
  Sum1/1 -> Out1/1
  Sum/1 -> Sum1/1
  In4/1 -> Derivative3/1
  In1/1 -> Derivative/1
  In2/1 -> Derivative1/1
  Constant/1 -> Product/2
  Product/1 -> Sum/2
  In3/1 -> Derivative2/1
  Constant1/1 -> Product1/2
  Product1/1 -> Sum/3

== system fullcar/Roll/Subsystem10 ==
  note: z
  note: fi
  note: theta
  note: z_p
  In1 : Inport
  In2 : Inport  Port=2
  In3 : Inport  Port=3
  In4 : Inport  Port=4
  Constant : Constant  Value=x_p
  Constant1 : Constant  Value=y_p
  Derivative{,1..3} (4 alike) : Derivative
  Product : Product  RndMeth=Zero
  Product1 : Product  RndMeth=Zero
  Sum1 : Sum
  Sum2 : Sum  Inputs=---
  Out1 : Outport
  wires:
  Derivative3/1 -> Sum2/3
  Derivative2/1 -> Product1/1
  Derivative1/1 -> Product/1
  Derivative/1 -> Sum1/1
  Constant1/1 -> Product1/2
  In3/1 -> Derivative2/1
  Constant/1 -> Product/2
  In2/1 -> Derivative1/1
  Sum1/1 -> Out1/1
  In1/1 -> Derivative/1
  Product/1 -> Sum2/1
  Product1/1 -> Sum2/2
  In4/1 -> Derivative3/1
  Sum2/1 -> Sum1/2

== system fullcar/Roll/Subsystem14 ==
  note: z_p
  note: theta
  note: fi
  note: z
  In1 : Inport
  In2 : Inport  Port=2
  In3 : Inport  Port=3
  In4 : Inport  Port=4
  Constant : Constant  Value=x_p
  Constant1 : Constant  Value=y_p
  Product : Product  RndMeth=Zero
  Product1 : Product  RndMeth=Zero
  Sum1 : Sum
  Sum2 : Sum  Inputs=---
  Out1 : Outport
  wires:
  Sum2/1 -> Sum1/2
  In4/1 -> Sum2/3
  Product1/1 -> Sum2/2
  Product/1 -> Sum2/1
  In1/1 -> Sum1/1
  Sum1/1 -> Out1/1
  In2/1 -> Product/1
  Constant/1 -> Product/2
  In3/1 -> Product1/1
  Constant1/1 -> Product1/2

== system fullcar/Roll/Subsystem2 ==
  note: z_2
  note: fi
  note: theta
  note: z
  In1 : Inport
  In2 : Inport  Port=2
  In3 : Inport  Port=3
  In4 : Inport  Port=4
  Constant : Constant  Value=b
  Constant1 : Constant  Value=w
  Derivative{,1..3} (4 alike) : Derivative
  Product : Product  RndMeth=Zero
  Product1 : Product  RndMeth=Zero
  Sum : Sum  Inputs=++-
  Sum1 : Sum  Inputs=+-
  Out1 : Outport
  wires:
  Derivative3/1 -> Sum1/2
  Derivative2/1 -> Product1/1
  Derivative1/1 -> Product/1
  Derivative/1 -> Sum/1
  Product1/1 -> Sum/3
  Constant1/1 -> Product1/2
  In3/1 -> Derivative2/1
  Product/1 -> Sum/2
  Constant/1 -> Product/2
  In2/1 -> Derivative1/1
  In1/1 -> Derivative/1
  In4/1 -> Derivative3/1
  Sum/1 -> Sum1/1
  Sum1/1 -> Out1/1

== system fullcar/Roll/Subsystem3 ==
  note: z
  note: theta
  note: fi
  note: z_3
  In1 : Inport
  In2 : Inport  Port=2
  In3 : Inport  Port=3
  In4 : Inport  Port=4
  Constant : Constant  Value=a
  Constant1 : Constant  Value=w
  Derivative{,1..3} (4 alike) : Derivative
  Product : Product  RndMeth=Zero
  Product1 : Product  RndMeth=Zero
  Sum : Sum  Inputs=++-
  Sum1 : Sum  Inputs=+-
  Out1 : Outport
  wires:
  Derivative3/1 -> Sum1/2
  Derivative2/1 -> Product1/1
  Derivative1/1 -> Product/1
  Derivative/1 -> Sum/1
  Sum1/1 -> Out1/1
  Sum/1 -> Sum1/1
  In4/1 -> Derivative3/1
  In1/1 -> Derivative/1
  In2/1 -> Derivative1/1
  Constant/1 -> Product/2
  Product/1 -> Sum/2
  In3/1 -> Derivative2/1
  Constant1/1 -> Product1/2
  Product1/1 -> Sum/3

== system fullcar/Roll/Subsystem4 ==
  note: z
  note: theta
  note: fi
  note: z_2
  In1 : Inport
  In2 : Inport  Port=2
  In3 : Inport  Port=3
  In4 : Inport  Port=4
  Constant : Constant  Value=b
  Constant1 : Constant  Value=w
  Product : Product  RndMeth=Zero
  Product1 : Product  RndMeth=Zero
  Sum : Sum  Inputs=+++
  Sum1 : Sum  Inputs=+-
  Out1 : Outport
  wires:
  Sum1/1 -> Out1/1
  Sum/1 -> Sum1/1
  In4/1 -> Sum1/2
  In1/1 -> Sum/1
  In2/1 -> Product/1
  Constant/1 -> Product/2
  Product/1 -> Sum/2
  In3/1 -> Product1/1
  Constant1/1 -> Product1/2
  Product1/1 -> Sum/3

== system fullcar/Roll/Subsystem5 ==
  note: z
  note: theta
  note: fi
  note: z_4
  In1 : Inport
  In2 : Inport  Port=2
  In3 : Inport  Port=3
  In4 : Inport  Port=4
  Constant : Constant  Value=b
  Constant1 : Constant  Value=w
  Derivative{,1..3} (4 alike) : Derivative
  Product : Product  RndMeth=Zero
  Product1 : Product  RndMeth=Zero
  Sum : Sum  Inputs=+-+
  Sum1 : Sum  Inputs=+-
  Out1 : Outport
  wires:
  Derivative3/1 -> Sum1/2
  Derivative2/1 -> Product1/1
  Derivative1/1 -> Product/1
  Derivative/1 -> Sum/1
  Sum1/1 -> Out1/1
  Sum/1 -> Sum1/1
  In4/1 -> Derivative3/1
  In1/1 -> Derivative/1
  In2/1 -> Derivative1/1
  Constant/1 -> Product/2
  Product/1 -> Sum/2
  In3/1 -> Derivative2/1
  Constant1/1 -> Product1/2
  Product1/1 -> Sum/3

== system fullcar/Roll/Subsystem6 ==
  note: z_3
  note: fi
  note: theta
  note: z
  In1 : Inport
  In2 : Inport  Port=2
  In3 : Inport  Port=3
  In4 : Inport  Port=4
  Constant : Constant  Value=a
  Constant1 : Constant  Value=w
  Product : Product  RndMeth=Zero
  Product1 : Product  RndMeth=Zero
  Sum : Sum  Inputs=++-
  Sum1 : Sum  Inputs=+-
  Out1 : Outport
  wires:
  Product1/1 -> Sum/3
  Constant1/1 -> Product1/2
  In3/1 -> Product1/1
  Product/1 -> Sum/2
  Constant/1 -> Product/2
  In2/1 -> Product/1
  In1/1 -> Sum/1
  In4/1 -> Sum1/2
  Sum/1 -> Sum1/1
  Sum1/1 -> Out1/1

== system fullcar/Roll/Subsystem9 ==
  note: z_4
  note: fi
  note: theta
  note: z
  In1 : Inport
  In2 : Inport  Port=2
  In3 : Inport  Port=3
  In4 : Inport  Port=4
  Constant : Constant  Value=b
  Constant1 : Constant  Value=w
  Product : Product  RndMeth=Zero
  Product1 : Product  RndMeth=Zero
  Sum : Sum  Inputs=+-+
  Sum1 : Sum  Inputs=+-
  Out1 : Outport
  wires:
  Product1/1 -> Sum/3
  Constant1/1 -> Product1/2
  In3/1 -> Product1/1
  Product/1 -> Sum/2
  Constant/1 -> Product/2
  In2/1 -> Product/1
  In1/1 -> Sum/1
  In4/1 -> Sum1/2
  Sum/1 -> Sum1/1
  Sum1/1 -> Out1/1

== system fullcar/system 1/Subsystem1 ==
  note: z_1
  note: q_1
  In1 : Inport
  In2 : Inport  Port=2
  Sum : Sum  Inputs=+-
  Out1 : Outport
  wires:
  In2/1 -> Sum/2
  In1/1 -> Sum/1
  Sum/1 -> Out1/1

== system fullcar/system 1/Subsystem2 ==
  note: q_1
  note: z_1
  In1 : Inport
  In2 : Inport  Port=2
  Derivative : Derivative
  Derivative1 : Derivative
  Sum : Sum  Inputs=+-
  Out1 : Outport
  wires:
  Sum/1 -> Out1/1
  In1/1 -> Derivative/1
  In2/1 -> Derivative1/1
  Derivative/1 -> Sum/1
  Derivative1/1 -> Sum/2

== system fullcar/system 1/Subsystem4 ==
  note: z
  note: theta
  note: fi
  note: z_1
  In1 : Inport
  In2 : Inport  Port=2
  In3 : Inport  Port=3
  In4 : Inport  Port=4
  Constant : Constant  Value=a
  Constant1 : Constant  Value=w
  Product : Product  RndMeth=Zero
  Product1 : Product  RndMeth=Zero
  Sum : Sum  Inputs=++-
  Sum1 : Sum  Inputs=+-
  Out1 : Outport
  wires:
  Sum1/1 -> Out1/1
  Sum/1 -> Sum1/1
  In4/1 -> Sum1/2
  In1/1 -> Sum/1
  In2/1 -> Product/1
  Constant/1 -> Product/2
  Product/1 -> Sum/2
  In3/1 -> Product1/1
  Constant1/1 -> Product1/2
  Product1/1 -> Sum/3

== system fullcar/system 1/Subsystem5 ==
  note: z_1
  note: fi
  note: theta
  note: z
  In1 : Inport
  In2 : Inport  Port=2
  In3 : Inport  Port=3
  In4 : Inport  Port=4
  Constant : Constant  Value=a
  Constant1 : Constant  Value=w
  Derivative{,1..3} (4 alike) : Derivative
  Product : Product  RndMeth=Zero
  Product1 : Product  RndMeth=Zero
  Sum : Sum  Inputs=++-
  Sum1 : Sum  Inputs=+-
  Out1 : Outport
  wires:
  Product1/1 -> Sum/3
  Constant1/1 -> Product1/2
  In3/1 -> Derivative2/1
  Product/1 -> Sum/2
  Constant/1 -> Product/2
  In2/1 -> Derivative1/1
  In1/1 -> Derivative/1
  In4/1 -> Derivative3/1
  Sum/1 -> Sum1/1
  Sum1/1 -> Out1/1
  Derivative/1 -> Sum/1
  Derivative1/1 -> Product/1
  Derivative2/1 -> Product1/1
  Derivative3/1 -> Sum1/2

== system fullcar/system 2/Subsystem1 ==
  note: q_2
  note: z_2
  In1 : Inport
  In2 : Inport  Port=2
  Sum : Sum  Inputs=+-
  Out1 : Outport
  wires:
  Sum/1 -> Out1/1
  In1/1 -> Sum/1
  In2/1 -> Sum/2

== system fullcar/system 2/Subsystem2 ==
  note: z_2
  note: q_2
  In1 : Inport
  In2 : Inport  Port=2
  Derivative : Derivative
  Derivative1 : Derivative
  Sum : Sum  Inputs=+-
  Out1 : Outport
  wires:
  Derivative1/1 -> Sum/2
  Derivative/1 -> Sum/1
  In2/1 -> Derivative1/1
  In1/1 -> Derivative/1
  Sum/1 -> Out1/1

== system fullcar/system 2/Subsystem5 ==
  note: z
  note: theta
  note: fi
  note: z_2
  In1 : Inport
  In2 : Inport  Port=2
  In3 : Inport  Port=3
  In4 : Inport  Port=4
  Constant : Constant  Value=b
  Constant1 : Constant  Value=w
  Derivative{,1..3} (4 alike) : Derivative
  Product : Product  RndMeth=Zero
  Product1 : Product  RndMeth=Zero
  Sum : Sum  Inputs=+--
  Sum1 : Sum  Inputs=+-
  Out1 : Outport
  wires:
  Sum1/1 -> Out1/1
  Sum/1 -> Sum1/1
  In4/1 -> Derivative3/1
  In1/1 -> Derivative/1
  In2/1 -> Derivative1/1
  Constant/1 -> Product/2
  Product/1 -> Sum/2
  In3/1 -> Derivative2/1
  Constant1/1 -> Product1/2
  Product1/1 -> Sum/3
  Derivative/1 -> Sum/1
  Derivative1/1 -> Product/1
  Derivative2/1 -> Product1/1
  Derivative3/1 -> Sum1/2

== system fullcar/system 2/Subsystem7 ==
  note: z_2
  note: fi
  note: theta
  note: z
  In1 : Inport
  In2 : Inport  Port=2
  In3 : Inport  Port=3
  In4 : Inport  Port=4
  Constant : Constant  Value=b
  Constant1 : Constant  Value=w
  Product : Product  RndMeth=Zero
  Product1 : Product  RndMeth=Zero
  Sum : Sum  Inputs=+--
  Sum1 : Sum  Inputs=+-
  Out1 : Outport
  wires:
  Product1/1 -> Sum/3
  Constant1/1 -> Product1/2
  In3/1 -> Product1/1
  Product/1 -> Sum/2
  Constant/1 -> Product/2
  In2/1 -> Product/1
  In1/1 -> Sum/1
  In4/1 -> Sum1/2
  Sum/1 -> Sum1/1
  Sum1/1 -> Out1/1

== system fullcar/system 3/Subsystem1 ==
  note: z_3
  note: q_3
  In1 : Inport
  In2 : Inport  Port=2
  Sum : Sum  Inputs=+-
  Out1 : Outport
  wires:
  In2/1 -> Sum/2
  In1/1 -> Sum/1
  Sum/1 -> Out1/1

== system fullcar/system 3/Subsystem10 ==
  note: z
  note: theta
  note: fi
  note: z_3
  In1 : Inport
  In2 : Inport  Port=2
  In3 : Inport  Port=3
  In4 : Inport  Port=4
  Constant : Constant  Value=a
  Constant1 : Constant  Value=w
  Product : Product  RndMeth=Zero
  Product1 : Product  RndMeth=Zero
  Sum : Sum  Inputs=+++
  Sum1 : Sum  Inputs=+-
  Out1 : Outport
  wires:
  Sum1/1 -> Out1/1
  Sum/1 -> Sum1/1
  In4/1 -> Sum1/2
  In1/1 -> Sum/1
  In2/1 -> Product/1
  Constant/1 -> Product/2
  Product/1 -> Sum/2
  In3/1 -> Product1/1
  Constant1/1 -> Product1/2
  Product1/1 -> Sum/3

== system fullcar/system 3/Subsystem2 ==
  note: q_3
  note: z_03
  In1 : Inport
  In2 : Inport  Port=2
  Derivative : Derivative
  Derivative1 : Derivative
  Sum : Sum  Inputs=+-
  Out1 : Outport
  wires:
  Sum/1 -> Out1/1
  In1/1 -> Derivative/1
  In2/1 -> Derivative1/1
  Derivative/1 -> Sum/1
  Derivative1/1 -> Sum/2

== system fullcar/system 3/Subsystem5 ==
  note: z_3
  note: fi
  note: theta
  note: z
  In1 : Inport
  In2 : Inport  Port=2
  In3 : Inport  Port=3
  In4 : Inport  Port=4
  Constant : Constant  Value=a
  Constant1 : Constant  Value=w
  Derivative{,1..3} (4 alike) : Derivative
  Product : Product  RndMeth=Zero
  Product1 : Product  RndMeth=Zero
  Sum : Sum  Inputs=+++
  Sum1 : Sum  Inputs=+-
  Out1 : Outport
  wires:
  Product1/1 -> Sum/3
  Constant1/1 -> Product1/2
  In3/1 -> Derivative2/1
  Product/1 -> Sum/2
  Constant/1 -> Product/2
  In2/1 -> Derivative1/1
  In1/1 -> Derivative/1
  In4/1 -> Derivative3/1
  Sum/1 -> Sum1/1
  Sum1/1 -> Out1/1
  Derivative/1 -> Sum/1
  Derivative1/1 -> Product/1
  Derivative2/1 -> Product1/1
  Derivative3/1 -> Sum1/2

== system fullcar/system 4/Subsystem1 ==
  note: q_4
  note: z_4
  In1 : Inport
  In2 : Inport  Port=2
  Sum : Sum  Inputs=+-
  Out1 : Outport
  wires:
  Sum/1 -> Out1/1
  In1/1 -> Sum/1
  In2/1 -> Sum/2

== system fullcar/system 4/Subsystem11 ==
  note: z
  note: theta
  note: fi
  note: z_4
  In1 : Inport
  In2 : Inport  Port=2
  In3 : Inport  Port=3
  In4 : Inport  Port=4
  Constant : Constant  Value=b
  Constant1 : Constant  Value=w
  Product : Product  RndMeth=Zero
  Product1 : Product  RndMeth=Zero
  Sum : Sum  Inputs=+-+
  Sum1 : Sum  Inputs=+-
  Out1 : Outport
  wires:
  Sum1/1 -> Out1/1
  Sum/1 -> Sum1/1
  In4/1 -> Sum1/2
  In1/1 -> Sum/1
  In2/1 -> Product/1
  Constant/1 -> Product/2
  Product/1 -> Sum/2
  In3/1 -> Product1/1
  Constant1/1 -> Product1/2
  Product1/1 -> Sum/3

== system fullcar/system 4/Subsystem2 ==
  note: z_04
  note: q_4
  In1 : Inport
  In2 : Inport  Port=2
  Derivative : Derivative
  Derivative1 : Derivative
  Sum : Sum  Inputs=+-
  Out1 : Outport
  wires:
  Derivative1/1 -> Sum/2
  Derivative/1 -> Sum/1
  In2/1 -> Derivative1/1
  In1/1 -> Derivative/1
  Sum/1 -> Out1/1

== system fullcar/system 4/Subsystem7 ==
  note: z_4
  note: fi
  note: theta
  note: z
  In1 : Inport
  In2 : Inport  Port=2
  In3 : Inport  Port=3
  In4 : Inport  Port=4
  Constant : Constant  Value=b
  Constant1 : Constant  Value=w
  Derivative{,1..3} (4 alike) : Derivative
  Product : Product  RndMeth=Zero
  Product1 : Product  RndMeth=Zero
  Sum : Sum  Inputs=+-+
  Sum1 : Sum  Inputs=+-
  Out1 : Outport
  wires:
  Product1/1 -> Sum/3
  Constant1/1 -> Product1/2
  In3/1 -> Derivative2/1
  Product/1 -> Sum/2
  Constant/1 -> Product/2
  In2/1 -> Derivative1/1
  In1/1 -> Derivative/1
  In4/1 -> Derivative3/1
  Sum/1 -> Sum1/1
  Sum1/1 -> Out1/1
  Derivative/1 -> Sum/1
  Derivative1/1 -> Product/1
  Derivative2/1 -> Product1/1
  Derivative3/1 -> Sum1/2

== system fullcar/system 5/Subsystem2 ==
  note: z_p
  note: theta
  note: fi
  note: z
  In1 : Inport
  In2 : Inport  Port=2
  In3 : Inport  Port=3
  In4 : Inport  Port=4
  Constant : Constant  Value=x_p
  Constant1 : Constant  Value=y_p
  Product : Product  RndMeth=Zero
  Product1 : Product  RndMeth=Zero
  Sum1 : Sum
  Sum2 : Sum  Inputs=---
  Out1 : Outport
  wires:
  Sum2/1 -> Sum1/2
  In4/1 -> Sum2/3
  Product1/1 -> Sum2/2
  Product/1 -> Sum2/1
  In1/1 -> Sum1/1
  Sum1/1 -> Out1/1
  In2/1 -> Product/1
  Constant/1 -> Product/2
  In3/1 -> Product1/1
  Constant1/1 -> Product1/2

== system fullcar/system 5/Subsystem3 ==
  note: z
  note: fi
  note: theta
  note: z_3
  In1 : Inport
  In2 : Inport  Port=2
  In3 : Inport  Port=3
  In4 : Inport  Port=4
  Constant : Constant  Value=x_p
  Constant1 : Constant  Value=y_p
  Derivative{,1..3} (4 alike) : Derivative
  Product : Product  RndMeth=Zero
  Product1 : Product  RndMeth=Zero
  Sum1 : Sum
  Sum2 : Sum  Inputs=---
  Out1 : Outport
  wires:
  Derivative3/1 -> Sum2/3
  Derivative2/1 -> Product1/1
  Derivative1/1 -> Product/1
  Derivative/1 -> Sum1/1
  Constant1/1 -> Product1/2
  In3/1 -> Derivative2/1
  Constant/1 -> Product/2
  In2/1 -> Derivative1/1
  Sum1/1 -> Out1/1
  In1/1 -> Derivative/1
  Product/1 -> Sum2/1
  Product1/1 -> Sum2/2
  In4/1 -> Derivative3/1
  Sum2/1 -> Sum1/2
